simulink model "Membrane_Distillation_R2023a"  (R2023a)
settings: Solver=VariableStepAuto  StartTime=0.0  StopTime=inf  RelTol=1e-3
settings Model: Creator=mekala.suresh  LastModifiedBy=andres.lucht
settings OptimizationCC: ReuseModelBlockBuffer=off

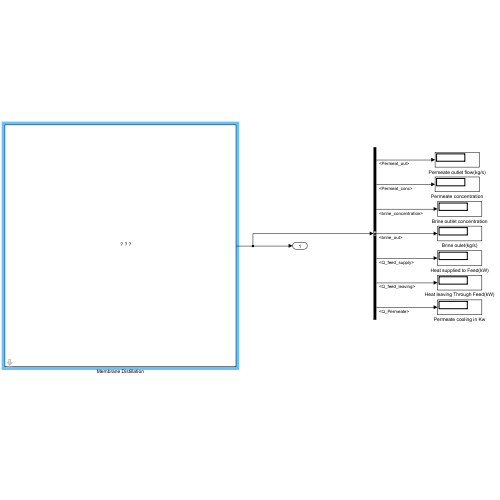
[thumbnail: Simulink's stored preview of the top-level diagram]
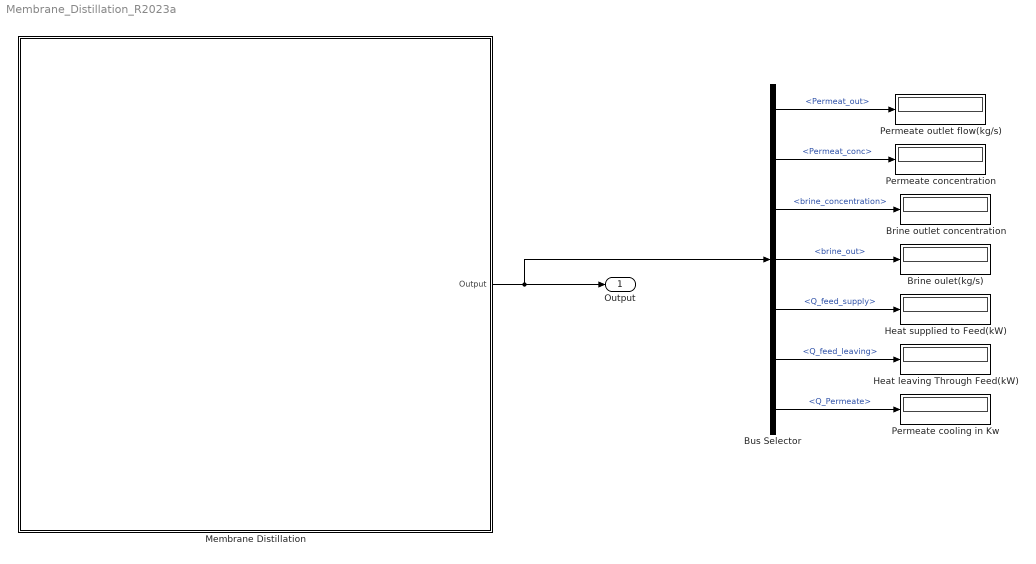
== system Membrane_Distillation_R2023a ==
  Brine oulet(kg/s) : Display
  Brine outlet concentration : Display
  Bus Selector : BusSelector  OutputSignals=Permeat_out,Permeat_conc,brine_concentration,brine_out,Q_feed_supply,Q_feed_leaving,Q_Permeate
  Heat leaving Through Feed(kW) : Display
  Heat supplied to Feed(kW) : Display
  Membrane Distillation : Subsystem  mask{T_feed=80, T_permeate=25, T_drop=020, T_mem=40, T_ambient=20, X_wf=0.965, X_Nacl=0.035, Inlet_flow=9, C_bf=35, P=151325, n=20, Diameter_of_Module=0.5, L=5, d_por=0.22e-6, delta=96e-6, epsilon=0.78, SR=0.9998}
      mask prompts: T_feed "Mean Feed Temeprature(°C)"; T_permeate "Mean Permeate Temperature(°C)"; T_drop "Temperature drop at outlet(°C)"; T_mem "Membrane Surface Temperature(°C)"; T_ambient "Ambinet Temperature(°C)"; X_wf "Mole fraction of water"; X_Nacl "Mole fraction of salt"; Inlet_flow "Inlet_flow(kg/s)"; C_bf "Bulk salt concentartion(kg/m3)"; P "Pressure (Pa)"; n "Number of modules"; Diameter_of_Module "Diameter of module(m)"; L "Length of Module(m)"; d_por "Pore diameters of Module(m)"; delta "Membrane thickness(m)"; epsilon "Membrane porosity(m)"; SR "Salt Rejection"
      mask DialogControl Container3 Prompt: Temperatures
      mask DialogControl Container4 Prompt: Inlet Flow Parameters
      mask DialogControl Container5 Prompt: Design Parameters
      mask DialogControl Container6 Prompt: Membrane Parameters
      mask Display: image('C:\Users\mekala.suresh\Desktop\Principle-of-the-membrane-distillation-MD-process.png'); % Use "Edit Image" on toolstrip to change.
  Permeate concentration : Display
  Permeate cooling in Kw : Display
  Permeate outlet flow(kg/s) : Display
  Output : Outport
  wires:
  Membrane Distillation/1(Output) -> Bus Selector/1, Output/1
  Bus Selector/1 -> Permeate outlet flow(kg/s)/1  "<Permeat_out>"
  Bus Selector/2 -> Permeate concentration/1  "<Permeat_conc>"
  Bus Selector/3 -> Brine outlet concentration/1  "<brine_concentration>"
  Bus Selector/4 -> Brine oulet(kg/s)/1  "<brine_out>"
  Bus Selector/5 -> Heat supplied to Feed(kW)/1  "<Q_feed_supply>"
  Bus Selector/6 -> Heat leaving Through Feed(kW)/1  "<Q_feed_leaving>"
  Bus Selector/7 -> Permeate cooling in Kw/1  "<Q_Permeate>"

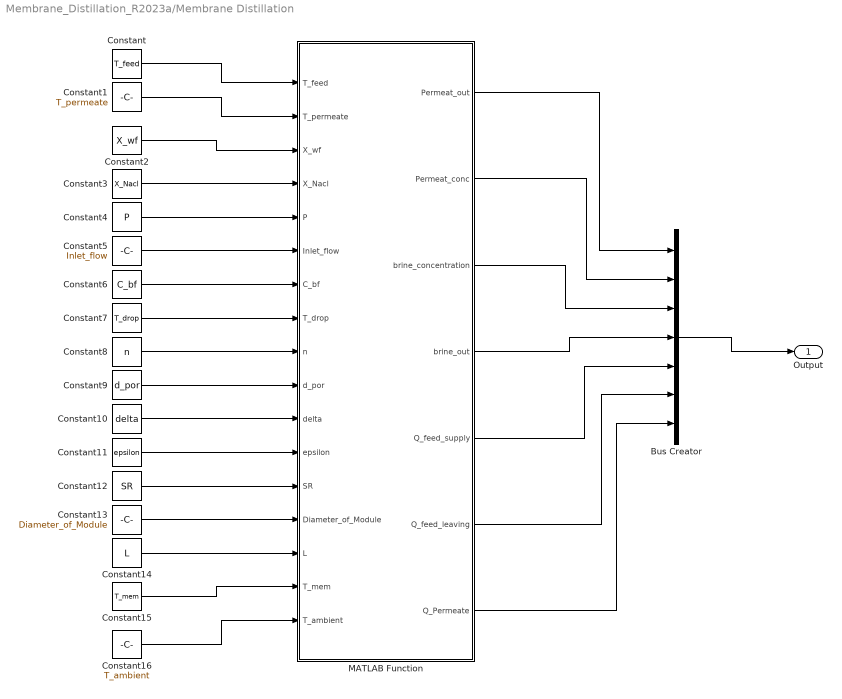
== system Membrane_Distillation_R2023a/Membrane Distillation ==
  Bus Creator : BusCreator  Inputs=7
  Constant : Constant  Value=T_feed
  Constant1 : Constant  Value=T_permeate
  Constant10 : Constant  Value=delta
  Constant11 : Constant  Value=epsilon
  Constant12 : Constant  Value=SR
  Constant13 : Constant  Value=Diameter_of_Module
  Constant14 : Constant  Value=L
  Constant15 : Constant  Value=T_mem
  Constant16 : Constant  Value=T_ambient
  Constant2 : Constant  Value=X_wf
  Constant3 : Constant  Value=X_Nacl
  Constant4 : Constant  Value=P
  Constant5 : Constant  Value=Inlet_flow
  Constant6 : Constant  Value=C_bf
  Constant7 : Constant  Value=T_drop
  Constant8 : Constant  Value=n
  Constant9 : Constant  Value=d_por
  MATLAB Function : MATLAB Function  TreatAsAtomicUnit=on
  Output : Outport
  wires:
  Constant6/1 -> MATLAB Function/7(C_bf)
  MATLAB Function/7(Q_Permeate) -> Bus Creator/7
  MATLAB Function/1(Permeat_out) -> Bus Creator/1
  Constant13/1 -> MATLAB Function/14(Diameter_of_Module)
  Constant5/1 -> MATLAB Function/6(Inlet_flow)
  MATLAB Function/3(brine_concentration) -> Bus Creator/3
  MATLAB Function/5(Q_feed_supply) -> Bus Creator/5
  Bus Creator/1 -> Output/1
  Constant7/1 -> MATLAB Function/8(T_drop)
  Constant9/1 -> MATLAB Function/10(d_por)
  Constant3/1 -> MATLAB Function/4(X_Nacl)
  Constant12/1 -> MATLAB Function/13(SR)
  MATLAB Function/6(Q_feed_leaving) -> Bus Creator/6
  MATLAB Function/2(Permeat_conc) -> Bus Creator/2
  Constant16/1 -> MATLAB Function/17(T_ambient)
  MATLAB Function/4(brine_out) -> Bus Creator/4
  Constant4/1 -> MATLAB Function/5(P)
  Constant15/1 -> MATLAB Function/16(T_mem)
  Constant/1 -> MATLAB Function/1(T_feed)
  Constant10/1 -> MATLAB Function/11(delta)
  Constant2/1 -> MATLAB Function/3(X_wf)
  Constant11/1 -> MATLAB Function/12(epsilon)
  Constant14/1 -> MATLAB Function/15(L)
  Constant8/1 -> MATLAB Function/9(n)
  Constant1/1 -> MATLAB Function/2(T_permeate)

== matlab function Membrane_Distillation_R2023a/Membrane Distillation/MATLAB Function ==
  data: T_feed input; Permeat_out output; T_permeate input; X_wf input; X_Nacl input; P input; Inlet_flow input; C_bf input; T_drop input; n input; d_por input; delta input; epsilon input; SR input; Diameter_of_Module input; L input; T_mem input; T_ambient input; Permeat_conc output; brine_concentration output; brine_out output; Q_feed_supply output; Q_feed_leaving output; Q_Permeate output
function [Permeat_out,Permeat_conc,brine_concentration,brine_out,Q_feed_supply,Q_feed_leaving,Q_Permeate] = fcn(T_feed,T_permeate,X_wf,X_Nacl,P,Inlet_flow,C_bf,T_drop,n,d_por,delta,epsilon,SR,Diameter_of_Module,L,T_mem,T_ambient)
%% Paper: Highly Saline Water Desalination Using Direct Contact Membrane Distillation (DCMD):
% Experimental and Simulation Study

% Copyright 2023 DECHEMA e.V., Theodor-Heuss-Allee 25, 60486 Frankfurt, Germany (https://dechema.de)
    % Contact: Andres Lucht Uribe
    % Developer: Suresh Mekala
    % Project H2Mare: https://www.wasserstoff-leitprojekte.de/projects/h2mare

%% Input System patrameters 

T_mf = T_feed+ 273;                          % feed mean temperature K
T_mp = T_permeate + 273;                     % permeate mean temperature K
R_g = 8.314;                                 % universal gas constant J/mol.K
M_wt =  18;                                  % total molecular weight of the water particle g/mol
%X_wf = 0.965;                               % water mole fraction in the feed water
%X_Nacl = 0.035;                             % Nacl mole fraction in the feed water
%P = 151325;                                 % P is the total pressure inside the pore (assumed to be constant and equal to the summation of the partial pressures of air and water)
%Inlet_flow = 5;                             % kg/sec
rho_l = 1000;                                % Density of liquid in hot channel                                  
mu = 0.001002;                               % viscosity of the fluid
%C_bf = 35;                                  % concentration of feed bulk kg/m3
%n = 20 ;                                    % Number of modules
T_amb = T_ambient+273;                       % Ambient Temperature K
C_p = 4180 ;                                 % Specific heat J/kg.K
%T_drop = 20 ;                                % Temperature drop K

%% Membrane properties

%d_por = 0.22e-6;                             % Diameter of pore m
%delta = 96e-6;                               % membrane thickness m
%epsilon = 0.78;                              % membrane porosity m
tau = ((2-epsilon)^2)/epsilon;                % membrane tortuosity
%SR = 0.9998;                                 % salt rejection rate

%% Design_Parameters 

%Diameter_of_Module = 0.5;                          % m
%L = 4;                                             % channel length m
CS_area =  ((pi/4)*(Diameter_of_Module^2));         % hot channel Cross_sectional_area for hydrolic diameter m2
wetted_peremeter = 2*pi*(Diameter_of_Module/2)*L;   % hot channel wetted_peremeter for hydrolic diameter m2
u = (Inlet_flow/1000)/CS_area;                      % Velocity of liquid in hot channel m/s

%% Partial Pressure calculations

T_m = ((T_mf+T_mp)/2);                       % mean temperature 
PD_WA = 1.895e-5 * (T_m^2.072);              % total pressure inside the pore * diffusion coefficent of air eq9
Pi = tau * delta;                            % membrane tortuosity
a_wf = 1 - (0.5*X_Nacl) -10*(X_Nacl^2) ;     % water activity coefficent
P_mf =exp(23.1964-(3816.44/(T_mf-46.13)));   % 
p_mf = P_mf* X_wf *a_wf;                     % eq6 partial pressure of water at the feed side
P_mp = exp(23.1964-(3816.44/(T_mp-46.13)));  % eq6 partial pressure of water at the permeate side

%% Diffusion coeffcient calculations

D_K =(((3*Pi)/(2*epsilon*d_por))*((pi*R_g*T_m)/((8*M_wt)))^0.5)^-1 ;  % eq7 Knudson diffusion coefficient
D_M = ((R_g*T_m*P*Pi)/(M_wt*epsilon*PD_WA))^-1;                       % eq8 Molecular diffusion coefficient
alphaa = D_K/D_M;                                                     % ratio of knudson diffusion to molecular diffusion (ranges 0-1)
D_e = ((alphaa/D_K)+((1-alphaa)/D_M))^-1;                             % eq7 Equivalent diffusion coefficent

%% Mass flux ;
% The mass flux in DCMD is proportional to the vapor pressure gradient through the membrane and can be given by the following equation
% Permeat flow and concentration

J = D_e*(p_mf-P_mp);                                        % eq1 Permeate mass flux g/m2.s
J_o = D_e *(p_mf - P_mp) *3.6;                              % eq1 Permeate mass flux kg/m2.h
Permeat_out = (J_o*wetted_peremeter*n)/3600;                % permeate outlet kg/sec 
Permeat_conc = (1-SR)*35;                                   % permeat concentration with salt rejection rate

%%  Polarization coefficent calculation  

D_h = (4*CS_area)/wetted_peremeter;                    % Hydrolic diameter
Re = (rho_l * u * D_h)/mu;                             % Reynolds number
Sc = mu / (rho_l * D_e);                               % Schmidt number
Sh = 1.86 * (Re * Sc * ((D_h / L)^(1 / 3)));           % Scherwood number
k_s =(Sh * D_e) / D_h ;                                % solute mass transfer coeffcient
C_mf = C_bf*exp(J/(k_s*rho_l));                        % Concnetration of solute at the membrane surface
POL_COEFF = C_mf/C_bf;                                 % Polarization coefficient

%% Brine flow & Cocentrations calculation

brine_out = Inlet_flow-Permeat_out;                                                     % brine outlet kg/sec 
brine_concentration = ((Inlet_flow*C_bf)-(Permeat_conc*Permeat_out))/brine_out;         % brine concentration computation

%% Power requirment calculations

T_lev = T_mf-T_drop;                                            % Brine leaving Temperature
%T_mem = 60+273;                                                % Temperature on the membrane side
Q_feed_supply = (Inlet_flow * C_p * (T_mf - T_amb))/1000;       % Heat supply to heat the feed flow to T_mf in KWatts
Q_feed_leaving = (brine_out * C_p * (T_lev - T_amb))/1000;      % Heat leaving with Brine Outlet_flow: T_lev in KWatts
Q_Permeate = (Permeat_out * C_p * (T_mem - T_mp))/1000;         % Cooling of Permeat flow in KWattts
